simulink model "tf_qPR"  (R2018b)
settings: Solver=ode23tb  StartTime=0.0  StopTime=10.0  RelTol=1e-3
values from neighbouring files (symbols this model uses):
  C = 5e-6    (= 5e-06)    [ziegler_nichols.m]
  kp = 0.1    [initialization.m]
  kr_1 = 100    [initialization.m]
  kr_3 = 100    [initialization.m]
  kr_5 = 100    [initialization.m]
  kr_7 = 100    [initialization.m]
  kr_9 = 100    [initialization.m]
  L = t(Tstart) - t(x_maxdStep)    [ziegler_nichols.m]
  rL = 0.1    [ziegler_nichols.m]
  w1 = 100*pi    (= 314.159265359)    [initialization.m]
  w3 = 100*pi*3    (= 942.477796077)    [initialization.m]
  w5 = 100*pi*5    (= 1570.79632679)    [initialization.m]
  w7 = 100*pi*7    (= 2199.11485751)    [initialization.m]
  w9 = 100*pi*9    (= 2827.43338823)    [initialization.m]
  wc = 5    [initialization.m]
settings Model: Creator=Xiaojie  LastModifiedBy=zxy49

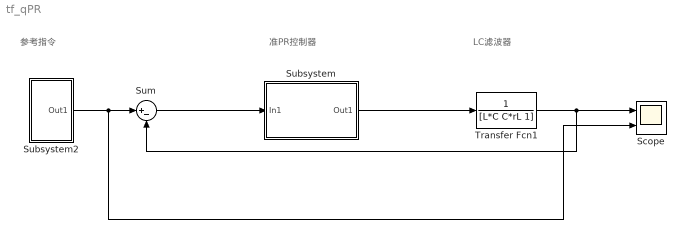
== system tf_qPR ==
  note: 准PR控制器
  note: LC滤波器
  note: 参考指令
  Scope : Scope  NumInputPorts=2
  Subsystem : Subsystem
  Subsystem2 : Subsystem
  Sum : Sum  Inputs=|+-
  Transfer Fcn1 : TransferFcn  Denominator=[L*C C*rL 1]
  wires:
  Sum/1 -> Subsystem/1(In1)
  Transfer Fcn1/1 -> Sum/2, Scope/1
  Subsystem2/1(Out1) -> Scope/2, Sum/1
  Subsystem/1(Out1) -> Transfer Fcn1/1

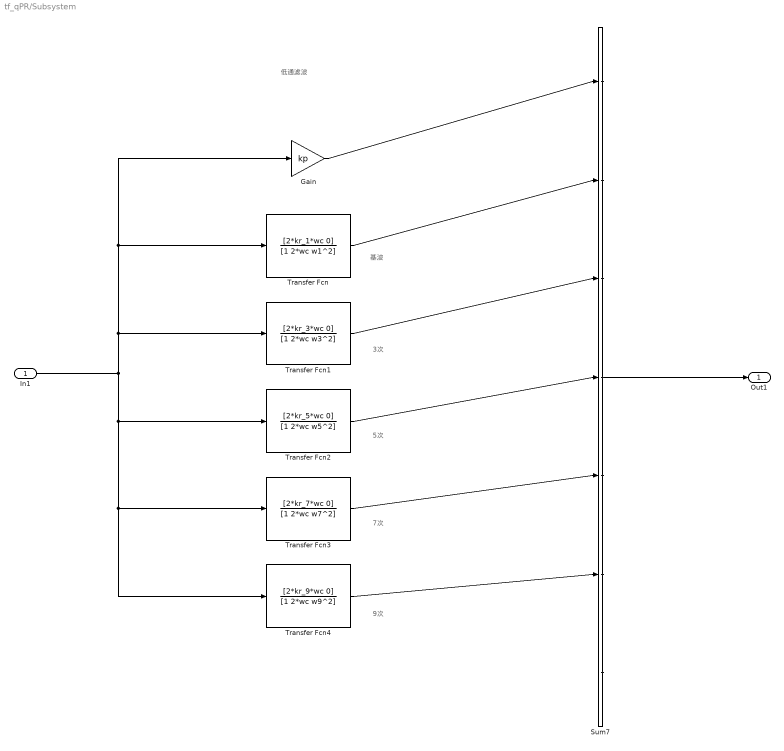
== system tf_qPR/Subsystem ==
  note: 基波
  note: 低通滤波
  note: 3次
  note: 5次
  note: 7次
  note: 9次
  In1 : Inport
  Gain : Gain  Gain=kp
  Sum7 : Sum  Inputs=|+++++++
  Transfer Fcn : TransferFcn  Numerator=[2*kr_1*wc 0]  Denominator=[1 2*wc w1^2]
  Transfer Fcn1 : TransferFcn  Numerator=[2*kr_3*wc 0]  Denominator=[1 2*wc w3^2]
  Transfer Fcn2 : TransferFcn  Numerator=[2*kr_5*wc 0]  Denominator=[1 2*wc w5^2]
  Transfer Fcn3 : TransferFcn  Numerator=[2*kr_7*wc 0]  Denominator=[1 2*wc w7^2]
  Transfer Fcn4 : TransferFcn  Numerator=[2*kr_9*wc 0]  Denominator=[1 2*wc w9^2]
  Out1 : Outport
  wires:
  Transfer Fcn4/1 -> Sum7/6
  Transfer Fcn1/1 -> Sum7/3
  In1/1 -> Transfer Fcn4/1, Transfer Fcn3/1, Transfer Fcn2/1, Transfer Fcn1/1, Gain/1, Transfer Fcn/1
  Transfer Fcn3/1 -> Sum7/5
  Transfer Fcn2/1 -> Sum7/4
  Gain/1 -> Sum7/1
  Transfer Fcn/1 -> Sum7/2
  Sum7/1 -> Out1/1

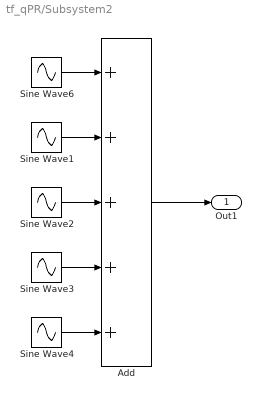
== system tf_qPR/Subsystem2 ==
  Add : Sum  Inputs=+++++
  Sine Wave1 : Sin  Amplitude=15  Frequency=2*pi*50*3  SampleTime=0
  Sine Wave2 : Sin  Amplitude=10  Frequency=2*pi*50*5  Phase=pi  SampleTime=0
  Sine Wave3 : Sin  Amplitude=10  Frequency=2*pi*50*7  Phase=pi  SampleTime=0
  Sine Wave4 : Sin  Amplitude=3  Frequency=2*pi*50*9  SampleTime=0
  Sine Wave6 : Sin  Amplitude=50  Frequency=2*pi*50*1  SampleTime=0
  Out1 : Outport
  wires:
  Sine Wave6/1 -> Add/1
  Add/1 -> Out1/1
  Sine Wave2/1 -> Add/3
  Sine Wave3/1 -> Add/4
  Sine Wave4/1 -> Add/5
  Sine Wave1/1 -> Add/2
